simulink library "INT_HPUn_QntBalInjLim"  (R2016b)
settings: Solver=VariableStepAuto  StartTime=0.0  StopTime=10.0  RelTol=1e-3
settings Model: Creator=Administrator  LastModifiedBy=Administrator

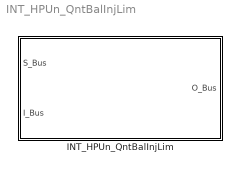
== system INT_HPUn_QntBalInjLim ==
  INT_HPUn_QntBalInjLim : Subsystem

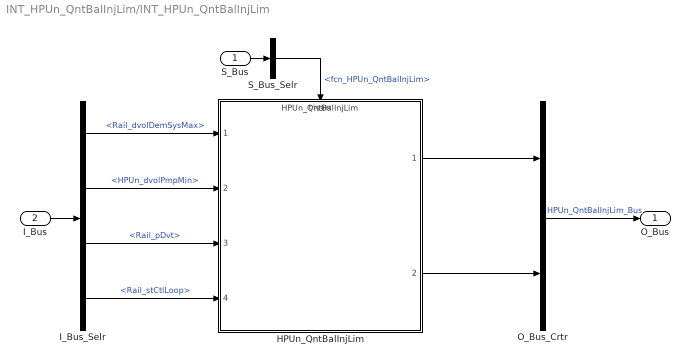
== system INT_HPUn_QntBalInjLim/INT_HPUn_QntBalInjLim ==
  S_Bus : Inport
  I_Bus : Inport  Port=2
  HPUn_QntBalInjLim : ModelReference  ModelNameDialog=HPUn_QntBalInjLim  SimulationMode=Normal  ModelReferenceVersion=1.18  TriggerPortName=function  TriggerPortTriggerType=function-call  TriggerPortStatesWhenEnabling=held
  I_Bus_Selr : BusSelector  OutputSignals=Rail_dvolDemSysMax,HPUn_dvolPmpMin,Rail_pDvt,Rail_stCtlLoop
  O_Bus_Crtr : BusCreator  Inputs=2
  S_Bus_Selr : BusSelector  OutputSignals=fcn_HPUn_QntBalInjLim
  O_Bus : Outport
  wires:
  S_Bus_Selr/1 -> HPUn_QntBalInjLim/Trigger  "<fcn_HPUn_QntBalInjLim>"
  S_Bus/1 -> S_Bus_Selr/1
  I_Bus/1 -> I_Bus_Selr/1
  I_Bus_Selr/1 -> HPUn_QntBalInjLim/1  "<Rail_dvolDemSysMax>"
  I_Bus_Selr/2 -> HPUn_QntBalInjLim/2  "<HPUn_dvolPmpMin>"
  I_Bus_Selr/3 -> HPUn_QntBalInjLim/3  "<Rail_pDvt>"
  I_Bus_Selr/4 -> HPUn_QntBalInjLim/4  "<Rail_stCtlLoop>"
  O_Bus_Crtr/1 -> O_Bus/1  "HPUn_QntBalInjLim_Bus"
  HPUn_QntBalInjLim/1 -> O_Bus_Crtr/1
  HPUn_QntBalInjLim/2 -> O_Bus_Crtr/2
